simulink model "blockdemo_18x18plus36"  (Simulink 7.6)
settings: Solver=ode45  StartTime=0.0  StopTime=100.0  RelTol=1e-3
InitFcn:
  | %% DSPBuilder Start
  | alt_dspbuilder_update_model(bdroot)
  | %% DSPBuilder End
libraries: allblocks_alteradspbuilder2 x6
settings Model: Creator=akarapet  LastModifiedBy=akarapet

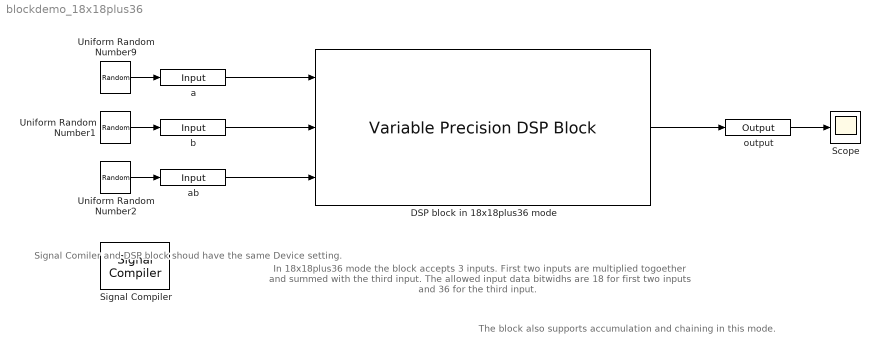
== system blockdemo_18x18plus36 ==
  note: In 18x18plus36 mode the block accepts 3 inputs.
      | First two inputs are multiplied togoether and summed
      | with the third input.
      | The allowed input data bitwidhs are 18 for first two inputs
      | and 36 for the third input.
  note: The block also supports accumulation and chaining in this mode.
  note: Signal Comiler and DSP block shoud
      | have the same Device setting.
  DSP block in 18x18plus36 mode : allblocks_alteradspbuilder2/Variable Precision DSP Block  complex_model_delayed=0  model_delayed=0  device_family=Arria V  used_mode_stratix=18x18+36 Mode  used_mode_arria=18x18+36 Mode  in_25x18_complex_mode=0  in_18x18plus36_mode=1  in_other_modes=0  number_of_mults=1  clock_ena_inputs=off  async_clear_inputs=off  bus_type=Signed Fractional  bwl_A=2  bwr_A=16  width_A=18  chain_width=64  reg_inputs_A=on  A_inputs_reg_ena=ENABLE 0  bwl_B=2  bwr_B=16  width_B=18  reg_inputs_B=on  B_inputs_reg_ena=ENABLE 0  bwl_joint_A_B=4  bwr_joint_A_B=32  reg_joint_A_B_input=on  A_B_input_reg_ena=ENABLE 0  bwl_A_complex=8  bwr_A_complex=8  reg_complex_A=on  A_complex_inputs_reg_ena=ENABLE 0  bwl_B_complex=8  bwr_B_complex=8  reg_complex_B=on  B_complex_inputs_reg_ena=ENABLE 0  A_inputs_exist=1  B_inputs_exist=1  C_inputs_exist=0  coef_sel_inputs_exist=0  all_inputs_registered=0  no_input_registered=0  all_inputs_share_same_clocks=0  full_resolution=off  bwl_out=5  bwr_out=32  reg_output=on  output_reg_ena=ENABLE 0  systolic_regs_available=0  enable_systolic_regs=off  systolic_regs_used=0  basic_struct_ok_for_input_scan=0  input_scan_available=0  enable_input_scan=off  input_scan_used=0  input_scan_delay_regs_available=0  enable_input_scan_delay_regs=off  input_scan_delay_regs_used=0  basic_struct_ok_for_coef_rom=0  coef_rom_available=0  enable_coef_rom=off  coef_rom_used=0  basic_struct_ok_for_preadder=0  preadder_available=0  enable_preadder=off  preadder_used=0  preadder_direction=ADD  square_mode_available=0  enable_square_mode=off  square_mode_used=0  upper_limit_9bit=9  upper_limit_18bit=19  upper_limit_27bit=27  in_18x18_modes=0  in_27x27_modes=0  in_36x18_modes=0  in_36x36_mode=0  mult1_adder_available=0  mult1_direction=ADD  mult3_adder_available=0  mult3_direction=ADD  chainout_adder_available=1  use_chainout_input=off  chainout_input_used=0  use_chainout_output=off  chainout_output_used=0  accum_available=1  enable_accum=off  accum_used=0  double_accum_available=0  enable_double_accum=off  double_accum_used=0  negate_available=1  mult_add_operation=ADD  rounding_constant_available=1  use_rounding_constant=off  rounding_constant_used=0  constant_value=1  bwl_C=8  bwr_C=0  bwl_coef=18  bwr_coef=0  mult0_coeffs=[0, 0, 0, 0, 0, 0, 0, 0]  mult1_coeffs=[0, 0, 0, 0, 0, 0, 0, 0]  mult2_coeffs=[0, 0, 0, 0, 0, 0, 0, 0]  mult3_coeffs=[0, 0, 0, 0, 0, 0, 0, 0]  reg_mult1_op_control=off  reg_mult3_op_control=off  reg_accum_control=off  reg_negate_control=off  control_regs_ena=ENABLE 0
  Scope : Scope
  Signal Compiler : allblocks_alteradspbuilder2/Signal Compiler  DeviceFamily=Arria V  DeviceName=AUTO  EnableSignalTap=off  SignalTapDepth=128  UseBoardBlock=off  StpUseDefaultClock=on  StpClock=Clock  ExportDir=<binary blob, 153 chars, not shown>
  Uniform Random Number1 : UniformRandomNumber  Minimum=-32000  Maximum=32000  Seed=345  SampleTime=1
  Uniform Random Number2 : UniformRandomNumber  Minimum=-9877765765  Maximum=233454556  Seed=222  SampleTime=1
  Uniform Random Number9 : UniformRandomNumber  Minimum=-32000  Maximum=32000  Seed=8889  SampleTime=1
  a : allblocks_alteradspbuilder2/Input  iofile=/data/akarapet/qshell_linux64_regtests/p4/dsp_builder/dsp_builder2/Documentation/DesignExamples/Tutorials/UnitBlocks/Arithmetic/VariablePrecisionDSPBlock/tb_blockdemo_18x18plus36/blockdemo%5F18x18plus36_a.salt  BusType=Signed Fractional  bwl=2  bwr=16  SpecifyClock=off  clock=default_clock  PORTTYPE=Input  externalType=Inferred  allowFloatingPointOverride=on  logOutputs=off
  ab : allblocks_alteradspbuilder2/Input  iofile=/data/akarapet/qshell_linux64_regtests/p4/dsp_builder/dsp_builder2/Documentation/DesignExamples/Tutorials/UnitBlocks/Arithmetic/VariablePrecisionDSPBlock/tb_blockdemo_18x18plus36/blockdemo%5F18x18plus36_ab.salt  BusType=Signed Fractional  bwl=4  bwr=32  SpecifyClock=off  clock=default_clock  PORTTYPE=Input  externalType=Inferred  allowFloatingPointOverride=on  logOutputs=off
  b : allblocks_alteradspbuilder2/Input  iofile=/data/akarapet/qshell_linux64_regtests/p4/dsp_builder/dsp_builder2/Documentation/DesignExamples/Tutorials/UnitBlocks/Arithmetic/VariablePrecisionDSPBlock/tb_blockdemo_18x18plus36/blockdemo%5F18x18plus36_b.salt  BusType=Signed Fractional  bwl=2  bwr=16  SpecifyClock=off  clock=default_clock  PORTTYPE=Input  externalType=Inferred  allowFloatingPointOverride=on  logOutputs=off
  output : allblocks_alteradspbuilder2/Output  iofile=/data/akarapet/qshell_linux64_regtests/p4/dsp_builder/dsp_builder2/Documentation/DesignExamples/Tutorials/UnitBlocks/Arithmetic/VariablePrecisionDSPBlock/tb_blockdemo_18x18plus36/blockdemo%5F18x18plus36_output.capture  BusType=Signed Fractional  bwl=5  bwr=32  externalType=Inferred  PORTTYPE=Output  allowFloatingPointOverride=on  logOutputs=off
  wires:
  Uniform Random Number9/1 -> a/1
  Uniform Random Number1/1 -> b/1
  Uniform Random Number2/1 -> ab/1
  a/1 -> DSP block in 18x18plus36 mode/1
  b/1 -> DSP block in 18x18plus36 mode/2
  ab/1 -> DSP block in 18x18plus36 mode/3
  DSP block in 18x18plus36 mode/1 -> output/1
  output/1 -> Scope/1
